simulink model "Lab3PartB"  (R2021b)
settings: Solver=ode45  StartTime=0.0  StopTime=15.5  RelTol=1e-3  EnableMultiTasking=on
libraries: simulink x1
settings Model: Creator=Kalai  LastModifiedBy=gajendrajayasekera
settings SolverCC: AlgebraicLoopSolver=TrustRegion
settings DataIOCC: LimitDataPoints=on  SaveFormat=Array  ReturnWorkspaceOutputs=off
settings OptimizationCC: LifeSpan=inf
settings DebuggingCC: UnderspecifiedInitializationDetection=Classic  MergeDetectMultiDrivingBlocksExec=none  SolverPrmCheckMsg=warning  SFUnexpectedBacktrackingDiag=warning  SFNoUnconditionalDefaultTransitionDiag=warning  SFExecutionAtInitializationDiag=none  SFMachineParentedDataDiag=warning  ArithmeticOperatorsInVariantConditions=warning
settings HardwareCC: ProdBitPerPointer=32  ProdBitPerSizeT=32  ProdBitPerPtrDiffT=32  ProdLargestAtomicFloat=None  ProdIntDivRoundTo=Undefined  ProdEndianess=Unspecified  ProdWordSize=32  ProdHWDeviceType=32-bit Generic
settings ModelReferenceCC: PropagateSignalLabelsOutOfModel=off
settings SFSimCC: SimUseLocalCustomCode=off  CustomCodeUndefinedFunction=UseInterfaceOnly
settings RTWCC: RTWUseLocalCustomCode=off
settings CodeAppCC: StateflowObjectComments=on
settings GRTTargetCC: TargetLangStandard=C89/C90 (ANSI)
settings ConfigComp: CovMetricSettings=dw  CovSaveCumulativeToWorkspaceVar=on  CovSaveSingleToWorkspaceVar=on  CovExternalEMLEnable=off

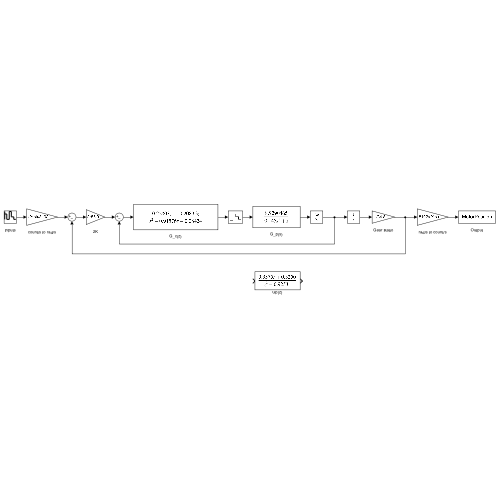
[thumbnail: Simulink's stored preview of the top-level diagram]
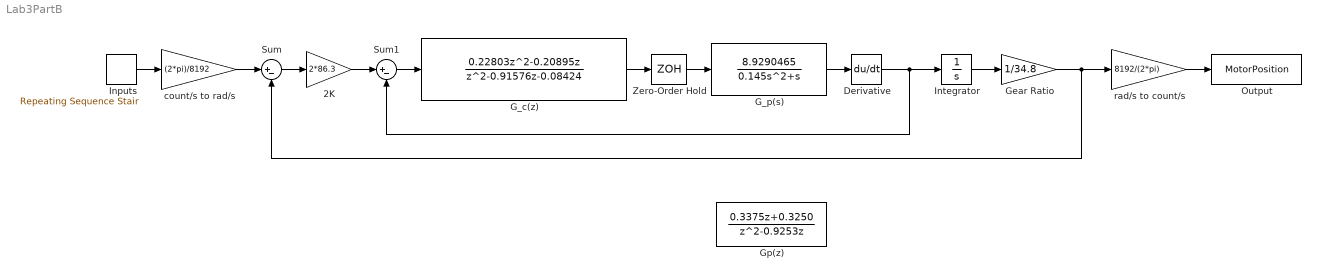
== system Lab3PartB ==
  " 2K" : Gain  Gain=2*86.3
  " G_c(z)" : DiscreteTransferFcn  Numerator=[0.22803 -0.20895 0]  Denominator=[1 -0.91576 -0.08424]  SampleTime=0.009
  " G_p(s)" : TransferFcn  Numerator=[8.9290465]  Denominator=[0.145 1 0]
  " Gear Ratio" : Gain  Gain=1/34.8
  " Inputs" : simulink/Sources/Repeating Sequence Stair  OutValues=|  tsamp=0.009  OutMin=[]  OutMax=[]  OutDataTypeStr=double  OutputDataTypeScalingMode=double  OutDataType=fixdt(0,8)  ConRadixGroup=Best Precision: Vector-wise  OutScaling=2^-12
      | [3072
      | 3072
      | 3072
      | 3072
      | 3072
      | 3072
      | 3072
      | 3072
      | 3072
      | 3072
      | 3072
      | 3072
      | 3072
      | 3072
      | 3072
      | 3072
      | 3072
      | 3072
      | 3072
      | 3072
      | 3072
      | 3072
      | 3072
      | 3072
      | 3072
      | 3072
      | 3072
      | 3072
      | 3072
      | 3072
      | 3072
      | 3072
      | 3072
      | 3072
      | 3072
      | 3072
      | 3072
      | 3072
      | 3072
      | 3072
      | 3072
      | 3072
      | 3072
      | 3072
      | 3072
      | 3072
      | 3072
      | 3072
      | 3072
      | 3072
      | 3072
      | 3072
      | 3072
      | 3072
      | 3072
      | 3072
      | 3072
      | 3072
      | 3072
      | 3072
      | 3072
      | 3072
      | 3072
      | 3072
      | 3072
      | 3072
      | 3072
      | 3072
      | 3072
      | 3072
      | 3072
      | 3072
      | 3072
      | 3072
      | 3072
      | 3072
      | 3072
      | 3072
      | 3072
      | 3072
      | 3072
      | 3072
      | 3072
      | 3072
      | 3072
      | 3072
      | 3072
      | 3072
      | 3072
      | 3072
      | 3072
      | 3072
      | 3072
      | 3072
      | 3072
      | 3072
      | 3072
      | 3072
      | 3072
      | 3072
      | 3072
      | 3072
      | 3072
      | 3072
      | 3072
      | 3072
      | 3072
      | 3072
      | 3072
      | 3072
      | 3072
      | 3072
      | 3072
      | 3072
      | 3072
      | 3072
      | 3072
      | 3072
      | 3072
      | 3072
      | 3072
      | 3072
      | 3072
      | 3072
      | 3072
      | 3072
      | 3072
      | 3072
      | 3072
      | 3072
      | 3072
      | 3072
      | 3072
      | 3072
      | 3072
      | 3072
      | 3072
      | 3072
      | 3072
      | 3072
      | 3072
      | 3072
      | 3072
      | 3072
      | 3072
      | 3072
      | 3072
      | 3072
      | 3072
      | 3072
      | 3072
      | 3072
      | 3072
      | 3072
      | 3072
      | 3072
      | 3072
      | 3072
      | 3072
      | 3072
      | 3072
      | 3072
      | 3072
      | 3072
      | 3072
      | 3072
      | 3072
      | 3072
      | 3072
      | 3072
      | 3072
      | 3072
      | 3072
      | 3072
      | 3072
      | 3072
      | 3072
      | 3072
      | 3072
      | 3072
      | 3072
      | 3072
      | 3072
      | 3072
      | 3072
      | 3072
      | 3072
      | 3072
      | 3072
      | 3072
      | 3072
      | 3072
      | 3072
      | 3072
      | 3072
      | 3072
      | 3072
      | 3072
      | 3072
      | 3072
      | 3072
      | 3072
      | 3072
      | 3072
      | 3072
      | 3072
      | 3072
      | 3072
      | 3072
      | 3072
      | 3072
      | 3072
      | 3072
      | 3072
      | 3072
      | 3072
      | 3072
      | 3072
      | 3072
      | 3072
      | 3072
      | 3072
      | 3072
      | 3072
      | 3072
      | 3072
      | 3072
      | 3072
      | 3072
      | 3072
      | 3072
      | 3072
      | 3072
      | 3072
      | 3072
      | 3072
      | 3072
      | 3072
      | 3072
      | 3072
      | 3072
      | 3072
      | 3072
      | 3072
      | 3072
      | 3072
      | 3072
      | 3072
      | 3072
      | 3072
      | 3072
      | 3072
      | 3072
      | 3072
      | 3072
      | 3072
      | 3072
      | 3072
      | 3072
      | 3072
      | 3072
      | 3072
      | 3072
      | 3072
      | 3072
      | 3072
      | 3072
      | 3072
      | 3072
      | 3072
      | 3072
      | 3072
      | 3072
      | 3072
      | 3072
      | 3072
      | 3072
      | 3072
      | 3072
      | 3072
      | 3072
      | 3072
      | 3072
      | 3072
      | 3072
      | 3072
      | 3072
      | 3072
      | 3072
      | 3072
      | 3072
      | 3072
      | 3072
      | 3072
      | 3072
      | 3072
      | 3072
      | 3072
      | 3072
      | 3072
      | 3072
      | 3072
      | 3072
      | 3072
      | 3072
      | 3072
      | 3072
      | 3072
      | 3072
      | 3072
      | 3072
      | 3072
      | 3072
      | 3072
      | 3072
      | 3072
      | 3072
      | 3072
      | 3072
      | 3072
      | 3072
      | 3072
      | 3072
      | 3072
      | 3072
      | 3072
      | 3072
      | 3072
      | 3072
      | 3072
      | 3072
      | 3072
      | 3072
      | 3072
      | 3072
      | 3072
      | 3072
      | 3072
      | 3072
      | 3072
      | 3072
      | 3072
      | 3072
      | 3072
      | 3072
      | 3072
      | 3072
      | 3072
      | 3072
      | 3072
      | 3072
      | 3072
      | 3072
      | 3072
      | 3072
      | 3072
      | 3072
      | 3072
      | 3072
      | 3072
      | 3072
      | 3072
      | 3072
      | 3072
      | 3072
      | 3072
      | 3072
      | 3072
      | 3072
      | 3072
      | 3072
      | 3072
      | 3072
      | 3072
      | 3072
      | 3072
      | 3072
      | 3072
      | 3072
      | 3072
      | 3072
      | 3072
      | 3072
      | 3072
      | 3072
      | 3072
      | 3072
      | 3072
      | 3072
      | 3072
      | 3072
      | 3072
      | 3072
      | 3072
      | 3072
      | 3072
      | 3072
      | 3072
      | 3072
      | 3072
      | 1024
      | 1024
      | 1024
      | 1024
      | 1024
      | 1024
      | 1024
      | 1024
      | 1024
      | 1024
      | 1024
      | 1024
      | 1024
      | 1024
      | 1024
      | 1024
      | 1024
      | 1024
      | 1024
      | 1024
      | 1024
      | 1024
      | 1024
      | 1024
      | 1024
      | 1024
      | 1024
      | 1024
      | 1024
      | 1024
      | 1024
      | 1024
      | 1024
      | 1024
      | 1024
      | 1024
      | 1024
      | 1024
      | 1024
      | 1024
      | 1024
      | 1024
      | 1024
      | 1024
      | 1024
      | 1024
      | 1024
      | 1024
      | 1024
      | 1024
      | 1024
      | 1024
      | 1024
      | 1024
      | 1024
      | 1024
      | 1024
      | 1024
      | 1024
      | 1024
      | 1024
      | 1024
      | 1024
      | 1024
      | 1024
      | 1024
      | 1024
      | 1024
      | 1024
      | 1024
      | 1024
      | 1024
      | 1024
      | 1024
      | 1024
      | 1024
      | 1024
      | 1024
      | 1024
      | 1024
      | 1024
      | 1024
      | 1024
      | 1024
      | 1024
      | 1024
      | 1024
      | 1024
      | 1024
      | 1024
      | 1024
      | 1024
      | 1024
      | 1024
      | 1024
      | 1024
      | 1024
      | 1024
      | 1024
      | 1024
      | 1024
      | 1024
      | 1024
      | 1024
      | 1024
      | 1024
      | 1024
      | 1024
      | 1024
      | 1024
      | 1024
      | 1024
      | 1024
      | 1024
      | 1024
      | 1024
      | 1024
      | 1024
      | 1024
      | 1024
      | 1024
      | 1024
      | 1024
      | 1024
      | 1024
      | 1024
      | 1024
      | 1024
      | 1024
      | 1024
      | 1024
      | 1024
      | 1024
      | 1024
      | 1024
      | 1024
      | 1024
      | 1024
      | 1024
      | 1024
      | 1024
      | 1024
      | 1024
      | 1024
      | 1024
      | 1024
      | 1024
      | 1024
      | 1024
      | 1024
      | 1024
      | 1024
      | 1024
      | 1024
      | 1024
      | 1024
      | 1024
      | 1024
      | 1024
      | 1024
      | 1024
      | 1024
      | 1024
      | 1024
      | 1024
      | 1024
      | 1024
      | 1024
      | 1024
      | 1024
      | 1024
      | 1024
      | 1024
      | 1024
      | 1024
      | 1024
      | 1024
      | 1024
      | 1024
      | 1024
      | 1024
      | 1024
      | 1024
      | 1024
      | 1024
      | 1024
      | 1024
      | 1024
      | 1024
      | 1024
      | 1024
      | 1024
      | 1024
      | 1024
      | 1024
      | 1024
      | 1024
      | 1024
      | 1024
      | 1024
      | 1024
      | 1024
      | 1024
      | 1024
      | 1024
      | 1024
      | 1024
      | 1024
      | 1024
      | 1024
      | 1024
      | 1024
      | 1024
      | 1024
      | 1024
      | 1024
      | 1024
      | 1024
      | 1024
      | 1024
      | 1024
      | 1024
      | 1024
      | 1024
      | 1024
      | 1024
      | 1024
      | 1024
      | 1024
      | 1024
      | 1024
      | 1024
      | 1024
      | 1024
      | 1024
      | 1024
      | 1024
      | 1024
      | 1024
      | 1024
      | 1024
      | 1024
      | 1024
      | 1024
      | 1024
      | 1024
      | 1024
      | 1024
      | 1024
      | 1024
      | 1024
      | 1024
      | 1024
      | 1024
      | 1024
      | 1024
      | 1024
      | 1024
      | 1024
      | 1024
      | 1024
      | 1024
      | 1024
      | 1024
      | 1024
      | 1024
      | 1024
      | 1024
      | 1024
      | 1024
      | 1024
      | 1024
      | 1024
      | 1024
      | 1024
      | 1024
      | 1024
      | 1024
      | 1024
      | 1024
      | 1024
      | 1024
      | 1024
      | 1024
      | 1024
      | 1024
      | 1024
      | 1024
      | 1024
      | 1024
      | 1024
      | 1024
      | 1024
      | 1024
      | 1024
      | 1024
      | 1024
      | 1024
      | 1024
      | 1024
      | 1024
      | 1024
      | 1024
      | 1024
      | 1024
      | 1024
      | 1024
      | 1024
      | 1024
      | 1024
      | 1024
      | 1024
      | 1024
      | 1024
      | 1024
      | 1024
      | 1024
      | 1024
      | 1024
      | 1024
      | 1024
      | 1024
      | 1024
      | 1024
      | 1024
      | 1024
      | 1024
      | 1024
      | 1024
      | 1024
      | 1024
      | 1024
      | 1024
      | 1024
      | 1024
      | 1024
      | 1024
      | 1024
      | 1024
      | 1024
      | 1024
      | 1024
      | 1024
      | 1024
      | 1024
      | 1024
      | 1024
      | 1024
      | 1024
      | 1024
      | 1024
      | 1024
      | 1024
      | 1024
      | 1024
      | 1024
      | 1024
      | 1024
      | 1024
      | 1024
      | 1024
      | 1024
      | 1024
      | 1024
      | 1024
      | 1024
      | 1024
      | 1024
      | 1024
      | 1024
      | 1024
      | 1024
      | 1024
      | 1024
      | 1024
      | 1024
      | 1024
      | 1024
      | 1024
      | 1024
      | 1024
      | 1024
      | 1024
      | 1024
      | 1024
      | 1024
      | 1024
      | 1024
      | 1024
      | 1024
      | 1024
      | 1024
      | 1024
      | 1024
      | 1024
      | 1024
      | 1024
      | 1024
      | 1024
      | 1024
      | 2048
      | 2048
      | 2048
      | 2048
      | 2048
      | 2048
      | 2048
      | 2048
      | 2048
      | 2048
      | 2048
      | 2048
      | 2048
      | 2048
      | 2048
      | 2048
      | 2048
      | 2048
      | 2048
      | 2048
      | 2048
      | 2048
      | 2048
      | 2048
      | 2048
      | 2048
      | 2048
      | 2048
      | 2048
      | 2048
      | 2048
      | 2048
      | 2048
      | 2048
      | 2048
      | 2048
      | 2048
      | 2048
      | 2048
      | 2048
      | 2048
      | 2048
      | 2048
      | 2048
      | 2048
      | 2048
      | 2048
      | 2048
      | 2048
      | 2048
      | 2048
      | 2048
      | 2048
      | 2048
      | 2048
      | 2048
      | 2048
      | 2048
      | 2048
      | 2048
      | 2048
      | 2048
      | 2048
      | 2048
      | 2048
      | 2048
      | 2048
      | 2048
      | 2048
      | 2048
      | 2048
      | 2048
      | 2048
      | 2048
      | 2048
      | 2048
      | 2048
      | 2048
      | 2048
      | 2048
      | 2048
      | 2048
      | 2048
      | 2048
      | 2048
      | 2048
      | 2048
      | 2048
      | 2048
      | 2048
      | 2048
      | 2048
      | 2048
      | 2048
      | 2048
      | 2048
      | 2048
      | 2048
      | 2048
      | 2048
      | 2048
      | 2048
      | 2048
      | 2048
      | 2048
      | 2048
      | 2048
      | 2048
      | 2048
      | 2048
      | 2048
      | 2048
      | 2048
      | 2048
      | 2048
      | 2048
      | 2048
      | 2048
      | 2048
      | 2048
      | 2048
      | 2048
      | 2048
      | 2048
      | 2048
      | 2048
      | 2048
      | 2048
      | 2048
      | 2048
      | 2048
      | 2048
      | 2048
      | 2048
      | 2048
      | 2048
      | 2048
      | 2048
      | 2048
      | 2048
      | 2048
      | 2048
      | 2048
      | 2048
      | 2048
      | 2048
      | 2048
      | 2048
      | 2048
      | 2048
      | 2048
      | 2048
      | 2048
      | 2048
      | 2048
      | 2048
      | 2048
      | 2048
      | 2048
      | 2048
      | 2048
      | 2048
      | 2048
      | 2048
      | 2048
      | 2048
      | 2048
      | 2048
      | 2048
      | 2048
      | 2048
      | 2048
      | 2048
      | 2048
      | 2048
      | 2048
      | 2048
      | 2048
      | 2048
      | 2048
      | 2048
      | 2048
      | 2048
      | 2048
      | 2048
      | 2048
      | 2048
      | 2048
      | 2048
      | 2048
      | 2048
      | 2048
      | 2048
      | 2048
      | 2048
      | 2048
      | 2048
      | 2048
      | 2048
      | 2048
      | 2048
      | 2048
      | 2048
      | 2048
      | 2048
      | 2048
      | 2048
      | 2048
      | 2048
      | 2048
      | 2048
      | 2048
      | 2048
      | 2048
      | 2048
      | 2048
      | 2048
      | 2048
      | 2048
      | 2048
      | 2048
      | 2048
      | 2048
      | 2048
      | 2048
      | 2048
      | 2048
      | 2048
      | 2048
      | 2048
      | 2048
      | 2048
      | 2048
      | 2048
      | 2048
      | 2048
      | 2048
      | 2048
      | 2048
      | 2048
      | 2048
      | 2048
      | 2048
      | 2048
      | 2048
      | 2048
      | 2048
      | 2048
      | 2048
      | 2048
      | 2048
      | 2048
      | 2048
      | 2048
      | 2048
      | 2048
      | 2048
      | 2048
      | 2048
      | 2048
      | 2048
      | 2048
      | 2048
      | 2048
      | 2048
      | 2048
      | 2048
      | 2048
      | 2048
      | 2048
      | 2048
      | 2048
      | 2048
      | 2048
      | 2048
      | 2048
      | 2048
      | 2048
      | 2048
      | 2048
      | 2048
      | 2048
      | 2048
      | 2048
      | 2048
      | 2048
      | 2048
      | 2048
      | 2048
      | 2048
      | 2048
      | 2048
      | 2048
      | 2048
      | 2048
      | 2048
      | 2048
      | 2048
      | 2048
      | 2048
      | 2048
      | 2048
      | 2048
      | 2048
      | 2048
      | 2048
      | 2048
      | 2048
      | 2048
      | 2048
      | 2048
      | 2048
      | 2048
      | 2048
      | 2048
      | 2048
      | 2048
      | 2048
      | 2048
      | 2048
      | 2048
      | 2048
      | 2048
      | 2048
      | 2048
      | 2048
      | 2048
      | 2048
      | 2048
      | 2048
      | 2048
      | 2048
      | 2048
      | 2048
      | 2048
      | 2048
      | 2048
      | 2048
      | 2048
      | 2048
      | 2048
      | 2048
      | 2048
      | 2048
      | 2048
      | 2048
      | 2048
      | 2048
      | 2048
      | 2048
      | 2048
      | 2048
      | 2048
      | 2048
      | 2048
      | 2048
      | 2048
      | 2048
      | 2048
      | 2048
      | 2048
      | 2048
      | 2048
      | 2048
      | 2048
      | 2048
      | 2048
      | 2048
      | 2048
      | 2048
      | 2048
      | 2048
      | 2048
      | 2048
      | 2048
      | 2048
      | 2048
      | 2048
      | 2048
      | 2048
      | 2048
      | 2048
      | 2048
      | 2048
      | 2048
      | 2048
      | 2048
      | 2048
      | 2048
      | 2048
      | 2048
      | 2048
      | 2048
      | 2048
      | 2048
      | 2048
      | 2048
      | 2048
      | 2048
      | 2048
      | 2560
      | 2560
      | 2560
      | 2560
      | 2560
      | 2560
      | 2560
      | 2560
      | 2560
      | 2560
      | 2560
      | 2560
      | 2560
      | 2560
      | 2560
      | 2560
      | 2560
      | 2560
      | 2560
      | 2560
      | 2560
      | 2560
      | 2560
      | 2560
      | 2560
      | 2560
      | 2560
      | 2560
      | 2560
      | 2560
      | 2560
      | 2560
      | 2560
      | 2560
      | 2560
      | 2560
      | 2560
      | 2560
      | 2560
      | 2560
      | 2560
      | 2560
      | 2560
      | 2560
      | 2560
      | 2560
      | 2560
      | 2560
      | 2560
      | 2560
      | 2560
      | 2560
      | 2560
      | 2560
      | 2560
      | 2560
      | 2560
      | 2560
      | 2560
      | 2560
      | 2560
      | 2560
      | 2560
      | 2560
      | 2560
      | 2560
      | 2560
      | 2560
      | 2560
      | 2560
      | 2560
      | 2560
      | 2560
      | 2560
      | 2560
      | 2560
      | 2560
      | 2560
      | 2560
      | 2560
      | 2560
      | 2560
      | 2560
      | 2560
      | 2560
      | 2560
      | 2560
      | 2560
      | 2560
      | 2560
      | 2560
      | 2560
      | 2560
      | 2560
      | 2560
      | 2560
      | 2560
      | 2560
      | 2560
      | 2560
      | 2560
      | 2560
      | 2560
      | 2560
      | 2560
      | 2560
      | 2560
      | 2560
      | 2560
      | 2560
      | 2560
      | 2560
      | 2560
      | 2560
      | 2560
      | 2560
      | 2560
      | 2560
      | 2560
      | 2560
      | 2560
      | 2560
      | 2560
      | 2560
      | 2560
      | 2560
      | 2560
      | 2560
      | 2560
      | 2560
      | 2560
      | 2560
      | 2560
      | 2560
      | 2560
      | 2560
      | 2560
      | 2560
      | 2560
      | 2560
      | 2560
      | 2560
      | 2560
      | 2560
      | 2560
      | 2560
      | 2560
      | 2560
      | 2560
      | 2560
      | 2560
      | 2560
      | 2560
      | 2560
      | 2560
      | 2560
      | 2560
      | 2560
      | 2560
      | 2560
      | 2560
      | 2560
      | 2560
      | 2560
      | 2560
      | 2560
      | 2560
      | 2560
      | 2560
      | 2560
      | 2560
      | 2560
      | 2560
      | 2560
      | 2560
      | 2560
      | 2560
      | 2560
      | 2560
      | 2560
      | 2560
      | 2560
      | 2560
      | 2560
      | 2560
      | 2560
      | 2560
      | 2560
      | 2560
      | 2560
      | 2560
      | 2560
      | 2560
      | 2560
      | 2560
      | 2560
      | 2560
      | 2560
      | 2560
      | 2560
      | 2560
      | 2560
      | 2560
      | 2560
      | 2560
      | 2560
      | 2560
      | 2560
      | 2560
      | 2560
      | 2560
      | 2560
      | 2560
      | 2560
      | 2560
      | 2560
      | 2560
      | 2560
      | 2560
      | 2560
      | 2560
      | 2560
      | 2560
      | 2560
      | 2560
      | 2560
      | 2560
      | 2560
      | 2560
      | 2560
      | 2560
      | 2560
      | 2560
      | 2560
      | 2560
      | 2560
      | 2560
      | 2560
      | 2560
      | 2560
      | 2560
      | 2560
      | 2560
      | 2560
      | 2560
      | 2560
      | 2560
      | 2560
      | 2560
      | 2560
      | 2560
      | 2560
      | 2560
      | 2560
      | 2560
      | 2560
      | 2560
      | 2560
      | 2560
      | 2560
      | 2560
      | 2560
      | 2560
      | 2560
      | 2560
      | 2560
      | 2560
      | 2560
      | 2560
      | 2560
      | 2560
      | 2560
      | 2560
      | 2560
      | 2560
      | 2560
      | 2560
      | 2560
      | 2560
      | 2560
      | 2560
      | 2560
      | 2560
      | 2560
      | 2560
      | 2560
      | 2560
      | 2560
      | 2560
      | 2560
      | 2560
      | 2560
      | 2560
      | 2560
      | 2560
      | 2560
      | 2560
      | 2560
      | 2560
      | 2560
      | 2560
      | 2560
      | 2560
      | 2560
      | 2560
      | 2560
      | 2560
      | 2560
      | 2560
      | 2560
      | 2560
      | 2560
      | 2560
      | 2560
      | 2560
      | 2560
      | 2560
      | 2560
      | 2560
      | 2560
      | 2560
      | 2560
      | 2560
      | 2560
      | 2560
      | 2560
      | 2560
      | 2560
      | 2560
      | 2560
      | 2560
      | 2560
      | 2560
      | 2560
      | 2560
      | 2560
      | 2560
      | 2560
      | 2560
      | 2560
      | 2560
      | 2560
      | 2560
      | 2560
      | 2560
      | 2560
      | 2560
      | 2560
      | 2560
      | 2560
      | 2560
      | 2560
      | 2560
      | 2560
      | 2560
      | 2560
      | 2560
      | 2560
      | 2560
      | 2560
      | 2560
      | 2560
      | 2560
      | 2560
      | 2560
      | 2560
      | 2560
      | 2560
      | 2560
      | 2560
      | 2560
      | 2560
      | 2560
      | 2560
      | 2560
      | 2560
      | 2560
      | 2560
      | 2560
      | 2560
      | 2560
      | 2560
      | 2560
      | 2560
      | 2560
      | 2560
      | 2560
      | 2560
      | 2560
      | 2560
      | 2560
      | 2560
      | 2560
      | 2560
      | 2560
      | 2560
      | 2560
      | 2560
      | 2560
      | 2560
      | 0
      | 0
      | 0
      | 0
      | 0
      | 0
      | 0
      | 0
      | 0
      | 0
      | 0
      | 0
      | 0
      | 0
      | 0
      | 0
      | 0
      | 0
      | 0
      | 0
      | 0
      | 0
      | 0
      | 0
      | 0
      | 0
      | 0
      | 0
      | 0
      | 0
      | 0
      | 0
      | 0
      | 0
      | 0
      | 0
      | 0
      | 0
      | 0
      | 0
      | 0
      | 0
      | 0
      | 0
      | 0
      | 0
      | 0
      | 0
      | 0
      | 0
      | 0
      | 0
      | 0
      | 0
      | 0
      | 0
      | 0
      | 0
      | 0
      | 0
      | 0
      | 0
      | 0
      | 0
      | 0
      | 0
      | 0
      | 0
      | 0
      | 0
      | 0
      | 0
      | 0
      | 0
      | 0
      | 0
      | 0
      | 0
      | 0
      | 0
      | 0
      | 0
      | 0
      | 0
      | 0
      | 0
      | 0
      | 0
      | 0
      | 0
      | 0
      | 0
      | 0
      | 0
      | 0
      | 0
      | 0
      | 0
      | 0
      | 0
      | 0
      | 0
      | 0
      | 0
      | 0
      | 0
      | 0
      | 0
      | 0
      | 0
      | 0
      | 0
      | 0
      | 0
      | 0
      | 0
      | 0
      | 0
      | 0
      | 0
      | 0
      | 0
      | 0
      | 0
      | 0
      | 0
      | 0
      | 0
      | 0
      | 0
      | 0
      | 0
      | 0
      | 0
      | 0
      | 0
      | 0
      | 0
      | 0
      | 0
      | 0
      | 0
      | 0
      | 0
      | 0
      | 0
      | 0
      | 0
      | 0
      | 0
      | 0
      | 0
      | 0
      | 0
      | 0
      | 0
      | 0
      | 0
      | 0
      | 0
      | 0
      | 0
      | 0
      | 0
      | 0
      | 0
      | 0
      | 0
      | 0
      | 0
      | 0
      | 0
      | 0
      | 0
      | 0
      | 0
      | 0
      | 0
      | 0
      | 0
      | 0
      | 0
      | 0
      | 0
      | 0
      | 0
      | 0
      | 0
      | 0
      | 0
      | 0
      | 0
      | 0
      | 0
      | 0
      | 0
      | 0
      | 0
      | 0
      | 0
      | 0
      | 0
      | 0
      | 0
      | 0
      | 0
      | 0
      | 0
      | 0
      | 0
      | 0
      | 0
      | 0
      | 0
      | 0
      | 0
      | 0
      | 0
      | 0
      | 0
      | 0
      | 0
      | 0
      | 0
      | 0
      | 0
      | 0
      | 0
      | 0
      | 0
      | 0
      | 0
      | 0
      | 0
      | 0
      | 0
      | 0
      | 0
      | 0
      | 0
      | 0
      | 0
      | 0
      | 0
      | 0
      | 0
      | 0
      | 0
      | 0
      | 0
      | 0
      | 0
      | 0
      | 0
      | 0
      | 0
      | 0
      | 0
      | 0
      | 0
      | 0
      | 0
      | 0
      | 0
      | 0
      | 0
      | 0
      | 0
      | 0
      | 0
      | 0
      | 0
      | 0
      | 0
      | 0
      | 0
      | 0
      | 0
      | 0
      | 0
      | 0
      | 0
      | 0
      | 0
      | 0
      | 0
      | 0
      | 0
      | 0
      | 0
      | 0
      | 0
      | 0
      | 0
      | 0
      | 0
      | 0
      | 0
      | 0
      | 0
      | 0
      | 0
      | 0
      | 0
      | 0
      | 0
      | 0
      | 0
      | 0
      | 0
      | 0
      | 0
      | 0
      | 0
      | 0
      | 0
      | 0
      | 0
      | 0
      | 0
      | 0
      | 0
      | 0
      | 0
      | 0
      | 0
      | 0
      | 0
      | 0
      | 0
      | 0
      | 0
      | 0
      | 0
      | 0
      | 0
      | 0
      | 0
      | 0
      | 0
      | 0
      | 0
      | 0
      | 0
      | 0
      | 0
      | 0
      | 0
      | 0
      | 0
      | 0
      | 0
      | 0
      | 0
      | 0
      | 0
      | 0
      | 0
      | 0
      | 0
      | 0
      | 0
      | 0
      | 0
      | 0
      | 0
      | 0
      | 0
      | 0
      | 0
      | 0
      | 0
      | 0
      | 0
      | 0
      | 0
      | 0
      | 0
      | 0
      | 0
      | 0
      | 0
      | 0
      | 0
      | 0
      | 0
      | 0
      | 0
      | 0
      | 0
      | 0
      | 0
      | 0
      | 0
      | 0
      | 0
      | 0
      | 0
      | 0
      | 0].'
  " Output" : ToWorkspace  VariableName=MotorPosition  SaveFormat=Timeseries  SampleTime=-1
  " count/s to rad/s" : Gain  Gain=(2*pi)/8192
  " rad/s to count/s" : Gain  Gain=8192/(2*pi)
  Derivative : Derivative
  Gp(z) : DiscreteTransferFcn  Numerator=[0.3375 0.3250]  Denominator=[1 -0.9253 0]  SampleTime=0.008
  Integrator : Integrator
  Sum : Sum  Inputs=|+-
  Sum1 : Sum  Inputs=|+-
  Zero-Order Hold : ZeroOrderHold  SampleTime=0.009
  wires:
  Sum/1 -> " 2K"/1
  " count/s to rad/s"/1 -> Sum/1
  " 2K"/1 -> Sum1/1
  Sum1/1 -> " G_c(z)"/1
  " G_c(z)"/1 -> Zero-Order Hold/1
  Zero-Order Hold/1 -> " G_p(s)"/1
  " G_p(s)"/1 -> Derivative/1
  Derivative/1 -> Integrator/1, Sum1/2
  Integrator/1 -> " Gear Ratio"/1
  " Gear Ratio"/1 -> " rad/s to count/s"/1, Sum/2
  " Inputs"/1 -> " count/s to rad/s"/1
  " rad/s to count/s"/1 -> " Output"/1
